simulink model "test"  (R2024b)
settings: Solver=ode45  StartTime=0.0  StopTime=1  MaxStep=0.0001  RelTol=1e-6
libraries: simulink_extras x8
settings Model: Creator=caohuaqi  LastModifiedBy=caohuaqi
settings DataIOCC: ExternalInput=[t]  InitialState=[]  LoadInitialState=on

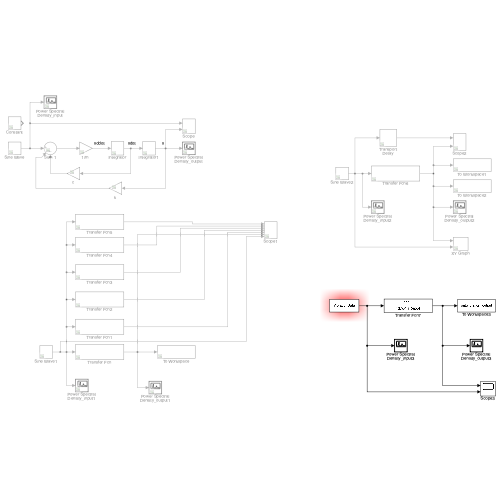
[thumbnail: Simulink's stored preview of the top-level diagram]
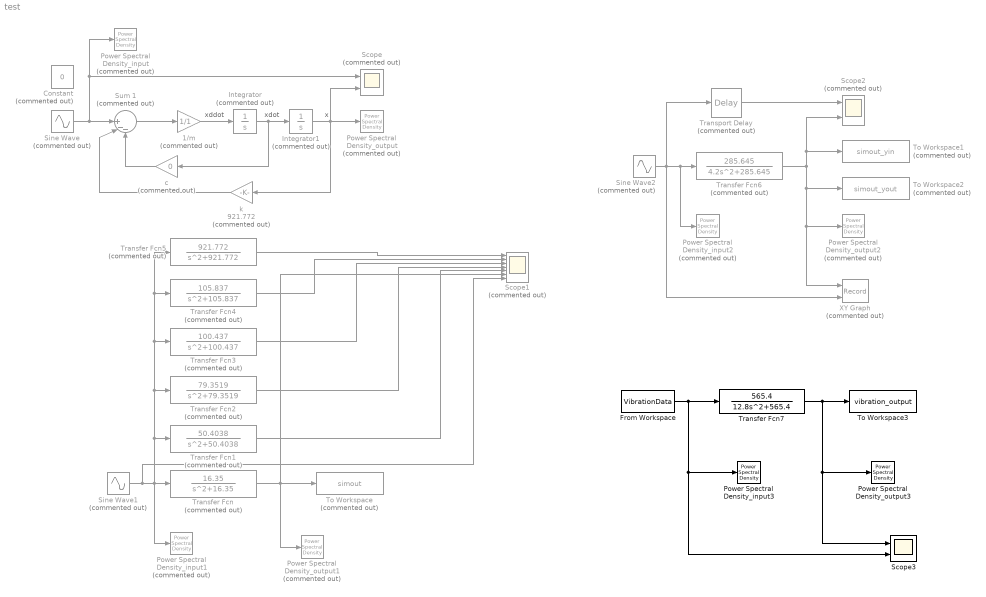
== system test ==
  note: x
  note: xdot
  note: xddot
  "1/m " : Gain  Commented=on  Gain=1/1
  Constant : Constant  Commented=on  Value=0
  From Workspace : FromWorkspace  VariableName=VibrationData
  Integrator : Integrator  Commented=on  IgnoreLimit=on
  Integrator1 : Integrator  Commented=on
  Power Spectral Density_input : simulink_extras/Additional Sinks/Power Spectral Density  Commented=on  npts=128  fftpts=512  HowOften=64  sampleT=0.1
  Power Spectral Density_input1 : simulink_extras/Additional Sinks/Power Spectral Density  Commented=on  npts=128  fftpts=512  HowOften=64  sampleT=0.1
  Power Spectral Density_input2 : simulink_extras/Additional Sinks/Power Spectral Density  Commented=on  npts=128  fftpts=512  HowOften=64  sampleT=0.1
  Power Spectral Density_input3 : simulink_extras/Additional Sinks/Power Spectral Density  npts=128  fftpts=512  HowOften=64  sampleT=0.1
  Power Spectral Density_output : simulink_extras/Additional Sinks/Power Spectral Density  Commented=on  npts=128  fftpts=512  HowOften=64  sampleT=0.1
  Power Spectral Density_output1 : simulink_extras/Additional Sinks/Power Spectral Density  Commented=on  npts=128  fftpts=512  HowOften=64  sampleT=0.1
  Power Spectral Density_output2 : simulink_extras/Additional Sinks/Power Spectral Density  Commented=on  npts=128  fftpts=512  HowOften=64  sampleT=0.1
  Power Spectral Density_output3 : simulink_extras/Additional Sinks/Power Spectral Density  npts=128  fftpts=512  HowOften=64  sampleT=0.1
  Scope : Scope  Commented=on  NumInputPorts=2
  Scope1 : Scope  Commented=on  NumInputPorts=7
  Scope2 : Scope  Commented=on  NumInputPorts=2
  Scope3 : Scope  NumInputPorts=2
  Sine Wave : Sin  Commented=on  Frequency=10  SampleTime=0
  Sine Wave1 : Sin  Commented=on  Frequency=10  SampleTime=0  VectorParams1D=off
  Sine Wave2 : Sin  Commented=on  Amplitude=0.01  Frequency=10  SampleTime=0  VectorParams1D=off
  Sum 1 : Sum  Commented=on  Inputs=||+--
  To Workspace : ToWorkspace  Commented=on  VariableName=simout  SaveFormat=Structure With Time
  To Workspace1 : ToWorkspace  Commented=on  VariableName=simout_yin  SaveFormat=Structure With Time
  To Workspace2 : ToWorkspace  Commented=on  VariableName=simout_yout  SaveFormat=Structure With Time
  To Workspace3 : ToWorkspace  VariableName=vibration_output  SaveFormat=Timeseries
      settings: MaxDataPoints=Inf
  Transfer Fcn : TransferFcn  Commented=on  Numerator=16.35  Denominator=[1 0 16.35]  ContinuousStateAttributes='position'
  Transfer Fcn1 : TransferFcn  Commented=on  Numerator=50.4038  Denominator=[1 0 50.4038]  ContinuousStateAttributes='position'
  Transfer Fcn2 : TransferFcn  Commented=on  Numerator=79.3519  Denominator=[1 0 79.3519]  ContinuousStateAttributes='position'
  Transfer Fcn3 : TransferFcn  Commented=on  Numerator=100.437  Denominator=[1 0 100.437]  ContinuousStateAttributes='position'
  Transfer Fcn4 : TransferFcn  Commented=on  Numerator=105.837  Denominator=[1 0 105.837]  ContinuousStateAttributes='position'
  Transfer Fcn5 : TransferFcn  Commented=on  Numerator=921.772  Denominator=[1 0 921.772]  ContinuousStateAttributes='position'
  Transfer Fcn6 : TransferFcn  Commented=on  Numerator=[0 285.645]  Denominator=[4.2 0 285.645]  ContinuousStateAttributes='position'
  Transfer Fcn7 : TransferFcn  Numerator=[0 565.4]  Denominator=[12.8 0 565.4]  ContinuousStateAttributes='position'
  Transport Delay : TransportDelay  Commented=on  DelayTime=0.157
  XY Graph : Record  Commented=on  FileSettingsInternal="{\"entries\":[{\"content\":{\"excelSettings\":{\"content\":{},\"type\":\"Streamout.ExcelSettings\"}},\"type\":\"Streamout.FileSettingStorage\",\"uuid\":\"\"}],\"packageUris\":[\"http:\\/\\/schema.mathworks.com\\/mf0\\/streamout_blocks\\/R2020a\"],\"version\":\"1.0\"}"  Layout=[1 1]  SignalsInternal="{\"entries\":[{\"content\":{\"signals\":[{\"content\":{\"blockPath\":[],\"dimensions\":[1,1],\"domain\":\"\",\"lineColor\":\"#77ac30\",\"lineWidth\":2,\"port\":1,\"signalID\":1,\"signalName\":\"Transfer Fcn6\"},\"type\":\"RecordBlkView.Signal\",\"uuid\":\"\"},{\"content\":{\"blockPath\":[],\"dimensions\":[1,1],\"domain\":\"\",\"lineColor\":\"#139fff\",\"plots\":[ 1 ],\"port\":2,\"signalID\":2,\"signalName\":\"Sine Wave2\"},\"type\":\"RecordBlkView.Signal\",\"uuid\":\"\"}]},\"type\":\"RecordBlkView.InputSignals\",\"uuid\":\"\"}],\"packageUris\":[\"http:\\/\\/schema.mathworks.com\\/mf0\\/streamout_blocks\\/R2020a\"],\"version\":\"1.0\"}"  VisualizationBindings="{\"xyplotplugin\":{\"info\":[{\"series\":[{\"bindingParametersList\":[{\"parameter\":\"Y-Axis\",\"signalID\":2,\"signalName\":\"Sine Wave2\"}],\"seriesID\":0}],\"subplotID\":1}]}}"  CompatibilityTag=XY
  c : Gain  Commented=on  Gain=0
  k : Gain  Commented=on  Gain=921.772
  wires:
  Integrator1/1 -> Power Spectral Density_output/1, Scope/2, k/1
  Integrator/1 -> c/1, Integrator1/1
  k/1 -> Sum 1/2
  c/1 -> Sum 1/3
  Sum 1/1 -> "1/m "/1
  "1/m "/1 -> Integrator/1
  Sine Wave/1 -> Sum 1/1, Scope/1, Power Spectral Density_input/1
  Sine Wave1/1 -> Scope1/7, Transfer Fcn1/1, Transfer Fcn5/1, Transfer Fcn4/1, Transfer Fcn3/1, Transfer Fcn2/1, Power Spectral Density_input1/1, Transfer Fcn/1
  Transfer Fcn/1 -> Power Spectral Density_output1/1, Scope1/6, To Workspace/1
  Transfer Fcn5/1 -> Scope1/1
  Transfer Fcn4/1 -> Scope1/2
  Transfer Fcn3/1 -> Scope1/3
  Transfer Fcn2/1 -> Scope1/4
  Transfer Fcn1/1 -> Scope1/5
  Transfer Fcn6/1 -> Scope2/2, To Workspace1/1, XY Graph/1, Power Spectral Density_output2/1, To Workspace2/1
  Sine Wave2/1 -> Transport Delay/1, XY Graph/2, Power Spectral Density_input2/1, Transfer Fcn6/1
  Transport Delay/1 -> Scope2/1
  Transfer Fcn7/1 -> Scope3/1, Power Spectral Density_output3/1, To Workspace3/1
  From Workspace/1 -> Scope3/2, Power Spectral Density_input3/1, Transfer Fcn7/1
